simulink model "sm_ball_bearing_testrig"  (R2026a)
settings: Solver=daessc  StopTime=10  MaxStep=1e-2  AbsTol=1e-3  EnableMultiTasking=on
PreLoadFcn:
  | sm_ball_bearing_testrig_param
StartFcn:
  | tic;
StopFcn:
  | Elapsed_Sim_Time = toc;
  | disp(['Elapsed Sim Time = ' num2str(Elapsed_Sim_Time)]);
undefined symbols (not defined in the file or in its folder): bearing, X, Y, Z
libraries: sm_lib x14, sm_ball_bearing_testrig_lib x2, nesl_utility x2
CloseFcn:
  | try,close(h1_sm_ball_bearing_testrig),end
  | clear h1_sm_ball_bearing_testrig
  | try,close(h2_sm_ball_bearing_testrig),end
  | clear h2_sm_ball_bearing_testrig
  | try,close(h3_sm_ball_bearing_testrig),end
  | clear h3_sm_ball_bearing_testrig
  | try,close(h4_sm_ball_bearing_testrig),end
  | clear h4_sm_ball_bearing_testrig
  | 
  | clear simlog_sm_ball_bearing_testrig
  | clear logsout_sm_ball_bearing_testrig
Description:
  | Ball Bearing Testrig
  | 
  | Copyright 2018-2026 The MathWorks, Inc.
settings Model: Creator=smiller  LastModifiedBy=smiller
settings DataIOCC: SignalLoggingName=logsout_sm_ball_bearing_testrig
settings DebuggingCC: PregeneratedLibrarySubsystemCodeDiagnostic=none
settings SimscapeCC: SimscapeNominalValues="[{\"value\":\"10\",\"unit\":\"V\"},{\"value\":\"1\",\"unit\":\"A\"},{\"value\":\"10\",\"unit\":\"N*m\"},{\"value\":\"10\",\"unit\":\"bar\"},{\"value\":\"100\",\"unit\":\"kJ/kg\"},{\"value\":\"1\",\"unit\":\"kW\"},{\"value\":\"300\",\"unit\":\"K\"},{\"value\":\"100\",\"unit\":\"cm^3/s\"},{\"value\":\"1\",\"unit\":\"kN\"},{\"value\":\"1\",\"unit\":\"g/cm^3\"},{\"value\":\"1\",\"unit\":\"l\"},{\"value\":\"1\",\"unit\":\"cm^2\"},{\"value\":\"60\",\"unit\":\"Hz\"}]"  SimscapeLogSimulationStatistics=on  SimscapeLogName=simlog_sm_ball_bearing_testrig
settings ConfigurationSet: Description=SimMechanics 2G
settings DiagnosticsConfigSet: SimMechanicsRigidlyBoundBlock=none
settings ExplorerConfigSet: InternalSimMechanicsExplorerSettings="<ExplorerConfiguration><canonicalview>default</canonicalview><AnimationSetting><BasePlaybackSpeed>1.0</BasePlaybackSpeed><PlaybackSpeedFactor>1.0</PlaybackSpeedFactor></AnimationSetting><TilePanel><TileInfo><Tiles Columns=\"1\" Count=\"1\" Rows=\"1\"><Column Weight=\"1\"/><Row Weight=\"1\"/><Tile Height=\"1\" Width=\"1\" X=\"0\" Y=\"0\"/></Tiles></TileInfo><SceneInfo><SceneViewer><BGColor><R>1</R><G>1</G><B>1</B></BGColor><Camera><DoPerspective>off</DoPerspective><Position><X>0.260257743485345527</X><Y>0.0410816638343565535</Y><Z>0.964664823166445862</Z></Position><Center><X>1.33669231247943751e-09</X><Y>-6.2585772627360983e-10</Y><Z>8.58219675317197067e-09</Z></Center><Up><X>-0.0188642502560075025</X><Y>0.999120072455301989</Y><Z>-0.0374595899495845999</Z></Up><ViewLimDist>1</ViewLimDist><YLim>0.0528120297938585309</YLim><XLim>0.0800932154702288929</XLim></Camera></SceneViewer></SceneInfo></TilePanel><MechEditorPanel><Cameras/><GfxPanelCameraMap/><VideoCreator><PlaybackSpeedRatio>1.0</PlaybackSpeedRatio><FrameRate>30</FrameRate><VideoFormat>Motion JPEG AVI</VideoFormat><FrameSize>auto</FrameSize></VideoCreator></MechEditorPanel></ExplorerConfiguration>"

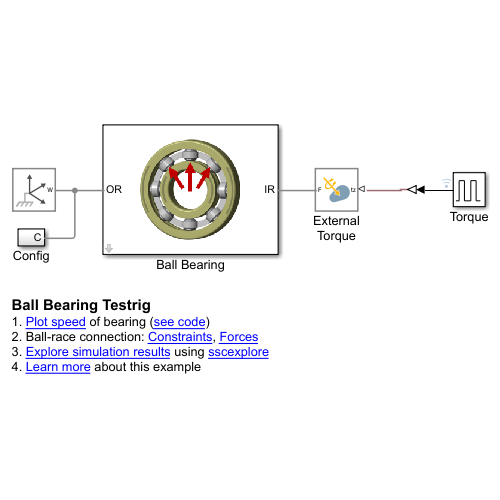
[thumbnail: Simulink's stored preview of the top-level diagram]
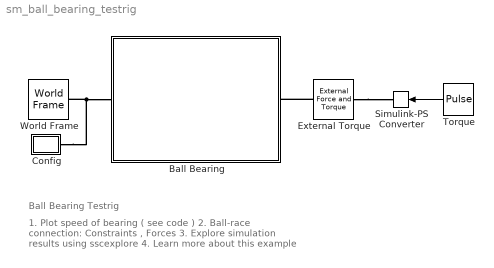
== system sm_ball_bearing_testrig ==
  note: Ball Bearing Testrig
  note: 1. Plot speed of bearing ( see code )
      | 2. Ball-race connection: Constraints , Forces
      | 3. Explore simulation results using sscexplore
      | 4. Learn more about this example
  Ball Bearing : Subsystem  Tag=PublishSubsystem  mask{bearing_or_xc=bearing.outer_race.xc, bearing_or_rho=bearing.outer_race.rho, bearing_or_clr=bearing.outer_race.clr, bearing_or_opc=bearing.outer_race.opc, bearing_or_mark_clr=bearing.outer_race.mark_clr, bearing_or_mark_opc=bearing.outer_race.mark_opc, bearing_or_mark_xc=bearing.outer_race.mark_xc, bearing_ir_xc=bearing.inner_race.xc, bearing_ir_rho=bearing.inner_race.rho, bearing_ir_clr=bearing.inner_race.clr, bearing_ir_opc=bearing.inner_race.opc, bearing_ir_mark_clr=bearing.inner_race.mark_clr, bearing_ir_mark_opc=bearing.inner_race.mark_opc, bearing_ir_mark_xc=bearing.inner_race.mark_xc, bearing_ball_rad=bearing.ball.rad, bearing_ball_rho=bearing.ball.rho, bearing_ball_cage_b=bearing.ball.cage_b, bearing_ball_clr=bearing.ball.clr, bearing_ball_opc=bearing.ball.opc, bearing_ball_mark_clr=bearing.ball.mark.clr, bearing_ball_mark_opc=bearing.ball.mark.opc, bearing_cage_loop_xc=bearing.cage.loop_xc, bearing_cage_web_xc=bearing.cage.web_xc, bearing_cage_web_thk=bearing.cage.thk, bearing_cage_rad_ctr=bearing.cage.web.centerrad, bearing_cage_rho=bearing.cage.rho, bearing_cage_clr=bearing.cage.clr, bearing_cage_opc=bearing.cage.opc, popup_constraints=Forces, bearing_ball_k=bearing.ball.k, bearing_ball_preload=bearing.ball.preload, bearing_ball_b=bearing.ball.b, bearing_ball_muk=bearing.ball.muk, bearing_ball_mus=bearing.ball.mus, bearing_ball_vth=bearing.ball.vth}
      mask prompts: bearing_or_xc "Cross Section in position [x y] (m)"; bearing_or_rho "Density (kg/m^3)"; bearing_or_clr "Color [R G B]"; bearing_or_opc "Opacity (0-1)"; bearing_or_mark_clr "Marking Color"; bearing_or_mark_opc "Marking Opacity (0-1)"; bearing_or_mark_xc "Marking Cross Section [x y] (m)"; bearing_ir_xc "Cross Section in position [x y] (m)"; bearing_ir_rho "Density (kg/m^3)"; bearing_ir_clr "Color [R G B]"; bearing_ir_opc "Opacity (0-1)"; bearing_ir_mark_clr "Marking Color"; bearing_ir_mark_opc "Marking Opacity (0-1)"; bearing_ir_mark_xc "Marking Cross Section [x y] (m)"; bearing_ball_rad "Radius (m)"; bearing_ball_rho "Density (kg/m^3)"; bearing_ball_cage_b "Ball-Cage Viscous Friction (N*m/(deg/s))"; bearing_ball_clr "Color [R G B]"; bearing_ball_opc "Opacity (0-1)"; bearing_ball_mark_clr "Marking Color [R G B]"; bearing_ball_mark_opc "Marking Opacity (0-1)"; bearing_cage_loop_xc "Cross Section for Loop [x y] (m)"; bearing_cage_web_xc "Cross Section for Web [x y] (m)"; bearing_cage_web_thk "Thickness of Web (m)"; bearing_cage_rad_ctr "Radius of Web Centerline (m)"; bearing_cage_rho "Density (kg/m^3)"; bearing_cage_clr "Color [RGB]"; bearing_cage_opc "Opacity"; popup_constraints "Connection"; bearing_ball_k "Stiffness (N/m)"; bearing_ball_preload "Preload Force Per Ball (N)"; bearing_ball_b "Damping (N/(m/s))"; bearing_ball_muk "Coefficient of Kinetic Friction"; bearing_ball_mus "Coefficient of Static Friction"; bearing_ball_vth "Velocity Threshold (m/s)"
      mask init:
      | if strcmp(get_param(gcb,'popup_constraints'),'Constraints')
      |     set_param([gcb '/Constrain Inner Outer'],'OverrideUsingVariant','Revolute');
      |     set_param([gcb '/Cage'],'OverrideUsingVariant','Constraints');
      | elseif strcmp(get_param(gcb,'popup_constraints'),'Forces')
      |     set_param([gcb '/Constrain Inner Outer'],'OverrideUsingVariant','Planar');
      |     set_param([gcb '/Cage'],'OverrideUsingVariant','Forces');
      | end
      mask TypeOptions popup_constraints: Constraints | Forces
      mask Callback popup_constraints:
      | maskObj = Simulink.Mask.get(gcb);
      | grf_h = maskObj.getDialogControl('group_frc');
      | if strcmp(get_param(gcb,'popup_constraints'),'Constraints')
      |     grf_h.Visible = 'off';
      | else
      |     grf_h.Visible = 'on';
      | end
      | clear maskObj grf_h
      mask DialogControl cont_or Prompt: Outer Race
      mask DialogControl cont_ir Prompt: Inner Race
      mask DialogControl cont_ball Prompt: Balls
      mask DialogControl cont_cage Prompt: Cage
      mask DialogControl cont_forces Prompt: Constraints
      mask Display:
      | if(strcmp(get_param(gcb,'popup_constraints'),'Constraints'))
      |     image('sm_ball_bearing_testrig_bearing_IMAGE.png')
      | else
      |     image('sm_ball_bearing_testrig_bearing_forces_IMAGE.png')
      | end
  Config : Subsystem
  External Torque : sm_lib/Forces and Torques/External Force and Torque  EnableForceX=off  EnableForceY=off  EnableForceZ=off  EnableForce=off  ForceResolutionFrame=AttachedFrame  EnableTorqueX=off  EnableTorqueY=off  EnableTorqueZ=on  EnableTorque=off  TorqueResolutionFrame=AttachedFrame
  Simulink-PS Converter : nesl_utility/Simulink-PS Converter  PhysicalDomain=network_engine_domain  SubClassName=ps_input  LeftPortType=input  RightPortType=output  PseudoPeriodic=off  Frequencies=[]  NoiseDistribution=none  NoiseParameters=[]  Unit=1  AffineConversion=off  FilteringAndDerivatives=provide  SimscapeFilterOrder=1  InputFilterTimeConstant=0.005  UdotUserProvided=0
  Torque : DiscretePulseGenerator  PulseType=Time based  Amplitude=-1e-3  Period=20  PulseWidth=5  PhaseDelay=1
  World Frame : sm_lib/Frames and Transforms/World Frame
  wires:
  Torque/1 -> Simulink-PS Converter/1
  connections:
  Config/RConn1 -- World Frame/RConn1 -- Ball Bearing/LConn1
  External Torque/LConn1 -- Simulink-PS Converter/RConn1
  External Torque/RConn1 -- Ball Bearing/RConn1

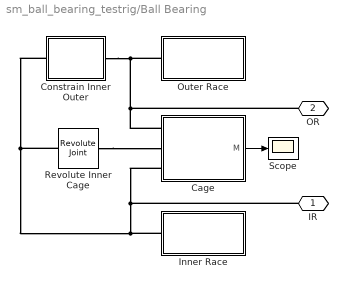
== system sm_ball_bearing_testrig/Ball Bearing ==
  Cage : Subsystem  Variant=on  VariantControlMode=label  VariantControl=Variant1  LabelModeActiveChoice=Forces
      mask Display:
      | blk = CFL_activeVariantBlock(gcb);
      | eval(get_param(blk, 'MaskDisplay'));
  Constrain Inner Outer : Subsystem  Variant=on  VariantControlMode=label  VariantControl=Variant1  LabelModeActiveChoice=Planar
      mask Display:
      | blk = CFL_activeVariantBlock(gcb);
      | eval(get_param(blk, 'MaskDisplay'));
  Inner Race : Subsystem  mask{ir_xc=bearing_ir_xc, ir_rho=bearing_ir_rho, ir_clr=bearing_ir_clr, ir_opc=bearing_ir_opc, ir_mark_clr=bearing_ir_mark_clr, ir_mark_opc=bearing_ir_mark_opc, ir_mark_xc=bearing_ir_mark_xc}
      mask prompts: ir_xc "Cross Section [x y] (m)"; ir_rho "Density (kg/m^3)"; ir_clr "Color [R G B]"; ir_opc "Opacity (0-1)"; ir_mark_clr "Marking Color"; ir_mark_opc "Marking Opacity (0-1)"; ir_mark_xc "Marking Cross Section [x y] (m)"
      mask DialogControl cont_ir Prompt: Inner Race
      mask Display: image('sm_ball_bearing_testrig_inner_race_IMAGE.png');
  Outer Race : Subsystem  Tag=PublishSubsystem  mask{or_xc=bearing_or_xc, or_rho=bearing_or_rho, or_clr=bearing_or_clr, or_opc=bearing_or_opc, or_mark_clr=bearing_or_mark_clr, or_mark_opc=bearing_or_mark_opc, or_mark_xc=bearing_or_mark_xc}
      mask prompts: or_xc "Cross Section [x y] (m)"; or_rho "Density (kg/m^3)"; or_clr "Color [R G B]"; or_opc "Opacity (0-1)"; or_mark_clr "Marking Color"; or_mark_opc "Marking Opacity (0-1)"; or_mark_xc "Marking Cross Section [x y] (m)"
      mask DialogControl cont_or Prompt: Outer Race
      mask Display: image('sm_ball_bearing_testrig_outer_race_IMAGE.png');
  Revolute Inner Cage : sm_lib/Joints/Revolute Joint  JointMode=Normal  CompositeWrenchDir=FollowerOnBase  CompositeWrenchFrame=BaseFrame  SenseConstraintForce=off  SenseConstraintTorque=off  SenseTotalForce=off  SenseTotalTorque=off  PositionTargetSpecify=off  PositionTargetPriority=High  PositionTargetValue=0  PositionTargetValueUnits=deg  VelocityTargetSpecify=off  VelocityTargetPriority=High  VelocityTargetValue=0  VelocityTargetValueUnits=deg/s  EquilibriumPosition=0  EquilibriumPositionUnits=deg  SpringStiffness=0  SpringStiffnessUnits=N*m/deg  DampingCoefficient=0  DampingCoefficientUnits=N*m/(deg/s)  LowerLimitSpecify=off  LowerLimitBound=-90  LowerLimitBoundUnits=deg  LowerLimitStiffness=1e4  LowerLimitStiffnessUnits=N*m/deg  LowerLimitDamping=10  LowerLimitDampingUnits=N*m/(deg/s)  LowerLimitTransitionRegionWidth=0.1  LowerLimitTransitionRegionWidthUnits=deg  UpperLimitSpecify=off  UpperLimitBound=90  UpperLimitBoundUnits=deg  UpperLimitStiffness=1e4  UpperLimitStiffnessUnits=N*m/deg  UpperLimitDamping=10  UpperLimitDampingUnits=N*m/(deg/s)  UpperLimitTransitionRegionWidth=0.1  UpperLimitTransitionRegionWidthUnits=deg  TorqueActuationMode=NoTorque  MotionActuationMode=ComputedMotion  SensePosition=off  SenseVelocity=off  SenseAcceleration=off  SenseTorqueForce=off  SenseLowerLimitTorqueForce=off  SenseUpperLimitTorqueForce=off
  Scope : Scope
      settings: ActiveDisplayYMinimum=4.08783  ActiveDisplayYMaximum=5.959
  IR : PMIOPort  Side=Right
  OR : PMIOPort  Port=2  Side=Left
  wires:
  Cage/1(M) -> Scope/1
  connections:
  Constrain Inner Outer/RConn1 -- OR/RConn1 -- Cage/LConn1 -- Outer Race/LConn1
  Inner Race/LConn1 -- Revolute Inner Cage/LConn1 -- Constrain Inner Outer/LConn1 -- IR/RConn1 -- Cage/LConn3
  Revolute Inner Cage/RConn1 -- Cage/LConn2

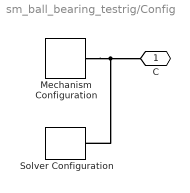
== system sm_ball_bearing_testrig/Config ==
  Mechanism Configuration : sm_lib/Utilities/Mechanism Configuration  UniformGravity=Constant  GravityVector=[0 -9.80665 0]  GravityVectorUnits=m/s^2  LinearizationDelta=0.001  JointModeTransitionNonlinearIterations=2
  Solver Configuration : nesl_utility/Solver Configuration  PhysicalDomain=network_engine_domain  SubClassName=solver  LeftPortType=input  RightPortType=generic  Tones=[]  Harmonics=[]  SimulateNoise=off  Profile=off  UseLocalSampling=off  EnableSwitchedLinearOptims=on  FrequencyDomain=off  UseCCode=off  RelTol=0.001  AbsTol=1e-06  MinStep=1e-09  ToWorkspace=off  RevertToSquareIcSolve=off  NumHomotopyIterations=100  PhasorMode=off  PhasorModeNumHarmonics=1  ConsistencySolver=NEWTON_FTOL  CanonicalOrdering=UNORDERED  OptimizeIntermediates=UNOPTIMIZED  IndexReductionMethod=DerivativeReplacement  DoDC=off  ResidualTolerance=1e-09  ConsistencyTolSource=GLOBAL  ConsistencyAbsTol=0.001  ConsistencyRelTol=0.001  ConsistencyTolFactor=0.001  UseLocalSolver=off  LocalSolverChoice=NE_BACKWARD_EULER_ADVANCER  ResolveIndetEquations=on  FunctionEvalNumThread=1  LocalSolverSampleTime=0.001  DoFixedCost=off  MaxNonlinIter=3  MaxModeIter=2  ComputeImpulses=off  ImpulseIterations=2  LinearAlgebra=Sparse  LinearAlgebraNumThread=0  EquationFormulation=NE_TIME_EF  DelaysMemoryBudget=1024  AutomaticFiltering=on  FilteringTimeConstant=0.001  PartitionStorageMethod=AS_NEEDED  PartitionMemoryBudget=1024  PartitionMethod=FAST  MultibodyUseLocalSolver=off  MultibodyLocalSolverChoice=ODE1  MultibodyLocalSolverSampleTime=0.001
  C : PMIOPort  Side=Right
  connections:
  Mechanism Configuration/RConn1 -- C/RConn1 -- Solver Configuration/RConn1

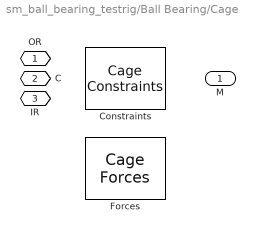
== system sm_ball_bearing_testrig/Ball Bearing/Cage ==
  Constraints : sm_ball_bearing_testrig_lib/Cage Constraints  Tag=PublishSubsystem  VariantControl=Constraints  ball_rad_all=bearing_ball_rad  ball_rho_all=bearing_ball_rho  ball_cage_b_all=bearing_ball_cage_b  ball_clr_all=bearing_ball_clr  ball_opc_all=bearing_ball_opc  ball_mark_clr_all=bearing_ball_mark_clr  ball_mark_opc_all=bearing_ball_mark_opc  bearing_or_all=max(bearing_or_xc(:,1))*2  bearing_ir_all=min(bearing_ir_xc(:,1))*2
  Forces : sm_ball_bearing_testrig_lib/Cage Forces  Tag=PublishSubsystem  VariantControl=Forces  ball_rad_all=bearing_ball_rad  ball_rho_all=bearing_ball_rho  ball_cage_b_all=bearing_ball_cage_b  ball_clr_all=bearing_ball_clr  ball_opc_all=bearing_ball_opc  ball_mark_clr_all=bearing_ball_mark_clr  ball_mark_opc_all=bearing_ball_mark_opc  bearing_or_all=max(bearing_or_xc(:,1))*2  bearing_ir_all=min(bearing_ir_xc(:,1))*2  ball_k_all=bearing_ball_k  ball_preload_all=bearing_ball_preload  ball_b_all=bearing_ball_b  ball_muk_all=bearing_ball_muk  ball_mus_all=bearing_ball_mus  ball_vth_all=bearing_ball_vth
  " OR " : PMIOPort  Side=Left
  " C " : PMIOPort  Port=2  Side=Left
  " IR " : PMIOPort  Port=3  Side=Left
  M : Outport  VectorParamsAs1DForOutWhenUnconnected=off

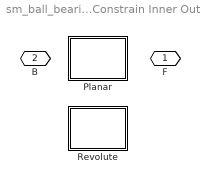
== system sm_ball_bearing_testrig/Ball Bearing/Constrain Inner Outer ==
  Planar : Subsystem  VariantControl=Planar
      mask Display: image('sm_ball_bearing_testrig_planar_IMAGE.png');
  Revolute : Subsystem  VariantControl=Revolute
      mask Display: image('sm_ball_bearing_testrig_revolute_IMAGE.png');
  " F " : PMIOPort  Side=Right
  " B " : PMIOPort  Port=2  Side=Left

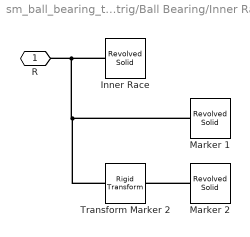
== system sm_ball_bearing_testrig/Ball Bearing/Inner Race ==
  Inner Race : sm_lib/Body Elements/Revolved Solid  RevolutionCrossSection=ir_xc  RevolutionCrossSectionUnits=m  RevolutionExtent=Full  RevolutionAngle=180  RevolutionAngleUnits=deg  ExportConvexHullGeometry=off  InertiaType=CalculateFromGeometry  BasedOnType=Density  Density=ir_rho  DensityUnits=kg/m^3  Mass=1  MassUnits=kg  CenterOfMass=[0 0 0]  CenterOfMassUnits=m  MomentsOfInertia=[1 1 1]  MomentsOfInertiaUnits=kg*m^2  ProductsOfInertia=[1 1 1]  ProductsOfInertiaUnits=kg*m^2  GraphicType=FromGeometry  MarkerShape=Sphere  MarkerSize=10  GraphicVisPropType=SimpleVisualProperties  GraphicDiffuseColor=ir_clr  GraphicOpacity=ir_opc  GraphicSpecularColor=[0.5 0.5 0.5 1.0]  GraphicAmbientColor=[0.15 0.15 0.15 1.0]  GraphicEmissiveColor=[0.0 0.0 0.0 1.0]  GraphicShininess=75  DoExposeReferenceFrame=on  SerializedFrames=<Frames/>
  Marker 1 : sm_lib/Body Elements/Revolved Solid  RevolutionCrossSection=ir_mark_xc  RevolutionCrossSectionUnits=m  RevolutionExtent=Custom  RevolutionAngle=60  RevolutionAngleUnits=deg  ExportConvexHullGeometry=off  InertiaType=CalculateFromGeometry  BasedOnType=Density  Density=0  DensityUnits=kg/m^3  Mass=1  MassUnits=kg  CenterOfMass=[0 0 0]  CenterOfMassUnits=m  MomentsOfInertia=[1 1 1]  MomentsOfInertiaUnits=kg*m^2  ProductsOfInertia=[1 1 1]  ProductsOfInertiaUnits=kg*m^2  GraphicType=FromGeometry  MarkerShape=Sphere  MarkerSize=10  GraphicVisPropType=SimpleVisualProperties  GraphicDiffuseColor=ir_mark_clr  GraphicOpacity=ir_mark_opc  GraphicSpecularColor=[0.5 0.5 0.5 1.0]  GraphicAmbientColor=[0.15 0.15 0.15 1.0]  GraphicEmissiveColor=[0.0 0.0 0.0 1.0]  GraphicShininess=75  DoExposeReferenceFrame=on  SerializedFrames=<Frames/>
  Marker 2 : sm_lib/Body Elements/Revolved Solid  RevolutionCrossSection=ir_mark_xc  RevolutionCrossSectionUnits=m  RevolutionExtent=Custom  RevolutionAngle=60  RevolutionAngleUnits=deg  ExportConvexHullGeometry=off  InertiaType=CalculateFromGeometry  BasedOnType=Density  Density=0  DensityUnits=kg/m^3  Mass=1  MassUnits=kg  CenterOfMass=[0 0 0]  CenterOfMassUnits=m  MomentsOfInertia=[1 1 1]  MomentsOfInertiaUnits=kg*m^2  ProductsOfInertia=[1 1 1]  ProductsOfInertiaUnits=kg*m^2  GraphicType=FromGeometry  MarkerShape=Sphere  MarkerSize=10  GraphicVisPropType=SimpleVisualProperties  GraphicDiffuseColor=ir_mark_clr  GraphicOpacity=ir_mark_opc  GraphicSpecularColor=[0.5 0.5 0.5 1.0]  GraphicAmbientColor=[0.15 0.15 0.15 1.0]  GraphicEmissiveColor=[0.0 0.0 0.0 1.0]  GraphicShininess=75  DoExposeReferenceFrame=on  SerializedFrames=<Frames/>
  Transform Marker 2 : sm_lib/Frames and Transforms/Rigid Transform  RotationMethod=StandardAxis  FollAlignAxisA=+X  BaseAlignAxisA=+Y  FollAlignAxisB=+Y  BaseAlignAxisB=+Z  RotationStandardAxis=+Z  RotationAngle=180  RotationAngleUnits=deg  RotationArbitraryAxis=[0 0 1]  RotationSequenceAxes=FollowerAxes  RotationSequence=XYX  RotationSequenceAngles=[0 0 0]  RotationSequenceAnglesUnits=deg  RotationMatrix=[1 0 0; 0 1 0; 0 0 1]  Quaternion=[1 0 0 0]  TranslationMethod=None  TranslationCartesianOffset=[0 0 0]  TranslationCartesianOffsetUnits=m  TranslationStandardAxis=+Z  TranslationStandardOffset=0  TranslationStandardOffsetUnits=m  TranslationROffset=0  TranslationROffsetUnits=m  TranslationThetaOffset=0  TranslationThetaOffsetUnits=deg  TranslationZOffset=0  TranslationZOffsetUnits=m
  R : PMIOPort  Side=Left
  connections:
  Marker 1/RConn1 -- R/RConn1 -- Inner Race/RConn1 -- Transform Marker 2/LConn1
  Marker 2/RConn1 -- Transform Marker 2/RConn1

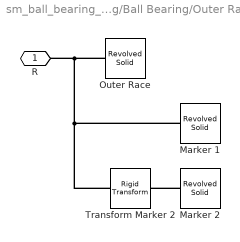
== system sm_ball_bearing_testrig/Ball Bearing/Outer Race ==
  Marker 1 : sm_lib/Body Elements/Revolved Solid  RevolutionCrossSection=or_mark_xc  RevolutionCrossSectionUnits=m  RevolutionExtent=Custom  RevolutionAngle=60  RevolutionAngleUnits=deg  ExportConvexHullGeometry=off  InertiaType=CalculateFromGeometry  BasedOnType=Density  Density=0  DensityUnits=kg/m^3  Mass=1  MassUnits=kg  CenterOfMass=[0 0 0]  CenterOfMassUnits=m  MomentsOfInertia=[1 1 1]  MomentsOfInertiaUnits=kg*m^2  ProductsOfInertia=[1 1 1]  ProductsOfInertiaUnits=kg*m^2  GraphicType=FromGeometry  MarkerShape=Sphere  MarkerSize=10  GraphicVisPropType=SimpleVisualProperties  GraphicDiffuseColor=or_mark_clr  GraphicOpacity=or_mark_opc  GraphicSpecularColor=[0.5 0.5 0.5 1.0]  GraphicAmbientColor=[0.15 0.15 0.15 1.0]  GraphicEmissiveColor=[0.0 0.0 0.0 1.0]  GraphicShininess=75  DoExposeReferenceFrame=on  SerializedFrames=<Frames/>
  Marker 2 : sm_lib/Body Elements/Revolved Solid  RevolutionCrossSection=or_mark_xc  RevolutionCrossSectionUnits=m  RevolutionExtent=Custom  RevolutionAngle=60  RevolutionAngleUnits=deg  ExportConvexHullGeometry=off  InertiaType=CalculateFromGeometry  BasedOnType=Density  Density=0  DensityUnits=kg/m^3  Mass=1  MassUnits=kg  CenterOfMass=[0 0 0]  CenterOfMassUnits=m  MomentsOfInertia=[1 1 1]  MomentsOfInertiaUnits=kg*m^2  ProductsOfInertia=[1 1 1]  ProductsOfInertiaUnits=kg*m^2  GraphicType=FromGeometry  MarkerShape=Sphere  MarkerSize=10  GraphicVisPropType=SimpleVisualProperties  GraphicDiffuseColor=or_mark_clr  GraphicOpacity=or_mark_opc  GraphicSpecularColor=[0.5 0.5 0.5 1.0]  GraphicAmbientColor=[0.15 0.15 0.15 1.0]  GraphicEmissiveColor=[0.0 0.0 0.0 1.0]  GraphicShininess=75  DoExposeReferenceFrame=on  SerializedFrames=<Frames/>
  Outer Race : sm_lib/Body Elements/Revolved Solid  RevolutionCrossSection=or_xc  RevolutionCrossSectionUnits=m  RevolutionExtent=Full  RevolutionAngle=180  RevolutionAngleUnits=deg  ExportConvexHullGeometry=off  InertiaType=CalculateFromGeometry  BasedOnType=Density  Density=or_rho  DensityUnits=kg/m^3  Mass=1  MassUnits=kg  CenterOfMass=[0 0 0]  CenterOfMassUnits=m  MomentsOfInertia=[1 1 1]  MomentsOfInertiaUnits=kg*m^2  ProductsOfInertia=[1 1 1]  ProductsOfInertiaUnits=kg*m^2  GraphicType=FromGeometry  MarkerShape=Sphere  MarkerSize=10  GraphicVisPropType=SimpleVisualProperties  GraphicDiffuseColor=or_clr  GraphicOpacity=or_opc  GraphicSpecularColor=[0.5 0.5 0.5 1.0]  GraphicAmbientColor=[0.15 0.15 0.15 1.0]  GraphicEmissiveColor=[0.0 0.0 0.0 1.0]  GraphicShininess=75  DoExposeReferenceFrame=on  SerializedFrames=<Frames/>
  Transform Marker 2 : sm_lib/Frames and Transforms/Rigid Transform  RotationMethod=StandardAxis  FollAlignAxisA=+X  BaseAlignAxisA=+Y  FollAlignAxisB=+Y  BaseAlignAxisB=+Z  RotationStandardAxis=+Z  RotationAngle=180  RotationAngleUnits=deg  RotationArbitraryAxis=[0 0 1]  RotationSequenceAxes=FollowerAxes  RotationSequence=XYX  RotationSequenceAngles=[0 0 0]  RotationSequenceAnglesUnits=deg  RotationMatrix=[1 0 0; 0 1 0; 0 0 1]  Quaternion=[1 0 0 0]  TranslationMethod=None  TranslationCartesianOffset=[0 0 0]  TranslationCartesianOffsetUnits=m  TranslationStandardAxis=+Z  TranslationStandardOffset=0  TranslationStandardOffsetUnits=m  TranslationROffset=0  TranslationROffsetUnits=m  TranslationThetaOffset=0  TranslationThetaOffsetUnits=deg  TranslationZOffset=0  TranslationZOffsetUnits=m
  R : PMIOPort  Side=Left
  connections:
  Outer Race/RConn1 -- Transform Marker 2/LConn1 -- Marker 1/RConn1 -- R/RConn1
  Marker 2/RConn1 -- Transform Marker 2/RConn1

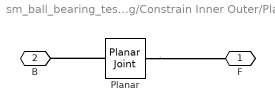
== system sm_ball_bearing_testrig/Ball Bearing/Constrain Inner Outer/Planar ==
  Planar : sm_lib/Joints/Planar Joint  JointMode=Normal  CompositeWrenchDir=FollowerOnBase  CompositeWrenchFrame=BaseFrame  SenseConstraintForce=off  SenseConstraintTorque=off  SenseTotalForce=off  SenseTotalTorque=off  PxPositionTargetSpecify=off  PxPositionTargetPriority=High  PxPositionTargetValue=0  PxPositionTargetValueUnits=m  PxVelocityTargetSpecify=off  PxVelocityTargetPriority=High  PxVelocityTargetValue=0  PxVelocityTargetValueUnits=m/s  PxEquilibriumPosition=0  PxEquilibriumPositionUnits=m  PxSpringStiffness=0  PxSpringStiffnessUnits=N/m  PxDampingCoefficient=0  PxDampingCoefficientUnits=N/(m/s)  PxLowerLimitSpecify=off  PxLowerLimitBound=-1  PxLowerLimitBoundUnits=m  PxLowerLimitStiffness=1e6  PxLowerLimitStiffnessUnits=N/m  PxLowerLimitDamping=1e3  PxLowerLimitDampingUnits=N/(m/s)  PxLowerLimitTransitionRegionWidth=1e-4  PxLowerLimitTransitionRegionWidthUnits=m  PxUpperLimitSpecify=off  PxUpperLimitBound=1  PxUpperLimitBoundUnits=m  PxUpperLimitStiffness=1e6  PxUpperLimitStiffnessUnits=N/m  PxUpperLimitDamping=1e3  PxUpperLimitDampingUnits=N/(m/s)  PxUpperLimitTransitionRegionWidth=1e-4  PxUpperLimitTransitionRegionWidthUnits=m  PxTorqueActuationMode=NoTorque  PxMotionActuationMode=ComputedMotion  PxSensePosition=off  PxSenseVelocity=off  PxSenseAcceleration=off  PxSenseTorqueForce=off  PxSenseLowerLimitTorqueForce=off  PxSenseUpperLimitTorqueForce=off  PyPositionTargetSpecify=off  PyPositionTargetPriority=High  PyPositionTargetValue=0  PyPositionTargetValueUnits=m  PyVelocityTargetSpecify=off  PyVelocityTargetPriority=High  PyVelocityTargetValue=0  PyVelocityTargetValueUnits=m/s  PyEquilibriumPosition=0  PyEquilibriumPositionUnits=m  PySpringStiffness=0  PySpringStiffnessUnits=N/m  PyDampingCoefficient=0  PyDampingCoefficientUnits=N/(m/s)  PyLowerLimitSpecify=off  PyLowerLimitBound=-1  PyLowerLimitBoundUnits=m  PyLowerLimitStiffness=1e6  PyLowerLimitStiffnessUnits=N/m  PyLowerLimitDamping=1e3  PyLowerLimitDampingUnits=N/(m/s)  PyLowerLimitTransitionRegionWidth=1e-4  PyLowerLimitTransitionRegionWidthUnits=m  PyUpperLimitSpecify=off  PyUpperLimitBound=1  PyUpperLimitBoundUnits=m  PyUpperLimitStiffness=1e6  PyUpperLimitStiffnessUnits=N/m  PyUpperLimitDamping=1e3  PyUpperLimitDampingUnits=N/(m/s)  PyUpperLimitTransitionRegionWidth=1e-4  PyUpperLimitTransitionRegionWidthUnits=m  PyTorqueActuationMode=NoTorque  PyMotionActuationMode=ComputedMotion  PySensePosition=off  PySenseVelocity=off  PySenseAcceleration=off  PySenseTorqueForce=off  PySenseLowerLimitTorqueForce=off  PySenseUpperLimitTorqueForce=off  RzPositionTargetSpecify=off  RzPositionTargetPriority=High  RzPositionTargetValue=0  RzPositionTargetValueUnits=deg  RzVelocityTargetSpecify=off  RzVelocityTargetPriority=High  RzVelocityTargetValue=0  RzVelocityTargetValueUnits=deg/s  RzEquilibriumPosition=0  RzEquilibriumPositionUnits=deg  RzSpringStiffness=0  RzSpringStiffnessUnits=N*m/deg  RzDampingCoefficient=0  RzDampingCoefficientUnits=N*m/(deg/s)  RzLowerLimitSpecify=off  RzLowerLimitBound=-90  RzLowerLimitBoundUnits=deg  RzLowerLimitStiffness=1e4  RzLowerLimitStiffnessUnits=N*m/deg  RzLowerLimitDamping=10  RzLowerLimitDampingUnits=N*m/(deg/s)  RzLowerLimitTransitionRegionWidth=0.1  RzLowerLimitTransitionRegionWidthUnits=deg  RzUpperLimitSpecify=off  RzUpperLimitBound=90  RzUpperLimitBoundUnits=deg  RzUpperLimitStiffness=1e4  RzUpperLimitStiffnessUnits=N*m/deg  RzUpperLimitDamping=10  RzUpperLimitDampingUnits=N*m/(deg/s)  RzUpperLimitTransitionRegionWidth=0.1  RzUpperLimitTransitionRegionWidthUnits=deg  RzTorqueActuationMode=NoTorque  RzMotionActuationMode=ComputedMotion  RzSensePosition=off  RzSenseVelocity=off  RzSenseAcceleration=off  RzSenseTorqueForce=off  RzSenseLowerLimitTorqueForce=off  RzSenseUpperLimitTorqueForce=off
  F : PMIOPort  Side=Right
  B : PMIOPort  Port=2  Side=Left
  connections:
  Planar/LConn1 -- B/RConn1
  Planar/RConn1 -- F/RConn1

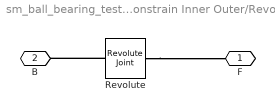
== system sm_ball_bearing_testrig/Ball Bearing/Constrain Inner Outer/Revolute ==
  Revolute : sm_lib/Joints/Revolute Joint  JointMode=Normal  CompositeWrenchDir=FollowerOnBase  CompositeWrenchFrame=BaseFrame  SenseConstraintForce=off  SenseConstraintTorque=off  SenseTotalForce=off  SenseTotalTorque=off  PositionTargetSpecify=off  PositionTargetPriority=High  PositionTargetValue=0  PositionTargetValueUnits=deg  VelocityTargetSpecify=off  VelocityTargetPriority=High  VelocityTargetValue=0  VelocityTargetValueUnits=deg/s  EquilibriumPosition=0  EquilibriumPositionUnits=deg  SpringStiffness=0  SpringStiffnessUnits=N*m/deg  DampingCoefficient=0  DampingCoefficientUnits=N*m/(deg/s)  LowerLimitSpecify=off  LowerLimitBound=-90  LowerLimitBoundUnits=deg  LowerLimitStiffness=1e4  LowerLimitStiffnessUnits=N*m/deg  LowerLimitDamping=10  LowerLimitDampingUnits=N*m/(deg/s)  LowerLimitTransitionRegionWidth=0.1  LowerLimitTransitionRegionWidthUnits=deg  UpperLimitSpecify=off  UpperLimitBound=90  UpperLimitBoundUnits=deg  UpperLimitStiffness=1e4  UpperLimitStiffnessUnits=N*m/deg  UpperLimitDamping=10  UpperLimitDampingUnits=N*m/(deg/s)  UpperLimitTransitionRegionWidth=0.1  UpperLimitTransitionRegionWidthUnits=deg  TorqueActuationMode=NoTorque  MotionActuationMode=ComputedMotion  SensePosition=off  SenseVelocity=off  SenseAcceleration=off  SenseTorqueForce=off  SenseLowerLimitTorqueForce=off  SenseUpperLimitTorqueForce=off
  F : PMIOPort  Side=Right
  B : PMIOPort  Port=2  Side=Left
  connections:
  Revolute/RConn1 -- F/RConn1
  Revolute/LConn1 -- B/RConn1
